simulink model "step3"  (R2018a)
settings: Solver=ode45  StartTime=0.0  StopTime=4  RelTol=1e-3
values from neighbouring files (symbols this model uses):
  Beta = 0    [step2.m]
  Friction = 22600    [step2.m]
  Inertia = 250000    [step2.m]
  Lambdam = 14.3522    [step2.m]
  Ld = 0.0035218    [step2.m]
  Lq = 0.0035218    [step2.m]
  Pole = 118    [step2.m]
  R = 58    [step2.m]
  Ro = 1.225    [step2.m]
  Rs = 0.05    [step2.m]
  Vw = 11.8    [step2.m]
undefined symbols (not defined in the file or in its folder): Cpmax, Lambda_opt, level, Ls, Ts
libraries: powerlib x18, peRmsMeasurement x8, peTransforms x2, simulink x2, powerlib_extras x1, simulink_extras x1
settings Model: Creator=Xinyi Zhang  LastModifiedBy=Xinyi Zhang

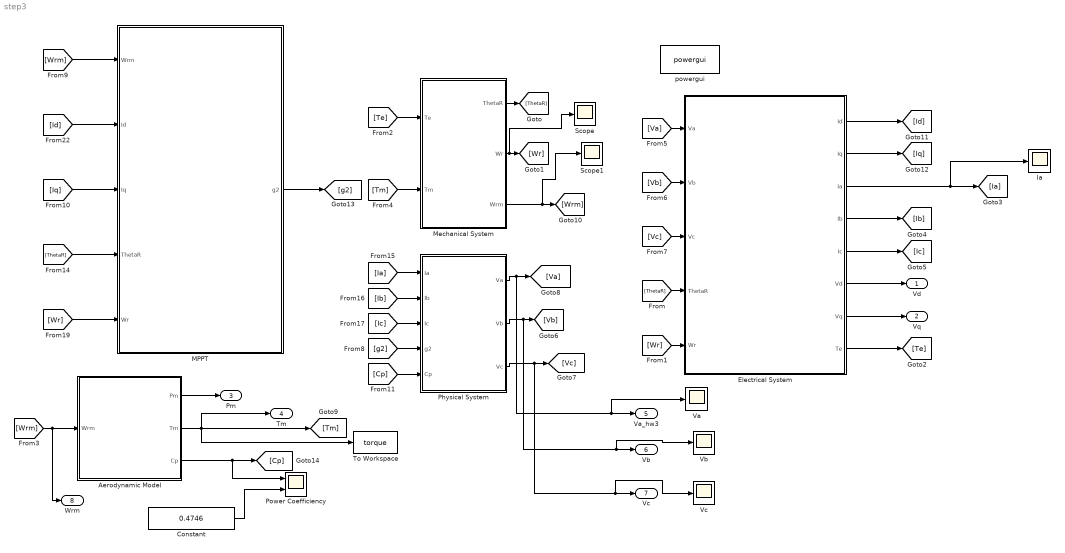
== system step3 ==
  "Aerodynamic Model " : Subsystem
  Constant : Constant  Value=0.4746
  "Electrical System " : Subsystem
  Ia : Scope
  "MPPT " : Subsystem
  "Mechanical System " : Subsystem
  "Physical System " : Subsystem
  "Power Coefficiency " : Scope  NumInputPorts=2
  Scope : Scope
  Scope1 : Scope
  To Workspace : ToWorkspace  VariableName=torque  SaveFormat=Timeseries  SampleTime=-1
  "Va " : Scope
  Vb : Scope
  Vc : Scope
  powergui : powerlib/powergui  Priority=1  SimulationMode=Discrete  SampleTime=25e-6  frequency=60  Iterations=50  frequencyindice=0  Pbase=100e6  ErrMax=1e-4  UnitsV=kV  UnitsW=MW  buscounter=0  FunctionMessages=off  echomessages=off  EnableUseOfTLC=off  CurrentSourceSwitches=off  DisableSnubberDevices=off  DisableRonSwitches=off  DisableVfSwitches=off  DisplayEquations=off  SolverType=Tustin/Backward Euler (TBE)  Interpol=off  ExternalGateDelay=off  methode=off  Ts=100  x0status=blocks  SPID=on  SwTol=0  HookPort=off  RestoreLinks=warning  ResistiveCurrentMeasurement=off  Frange=[0:2:500]  Ylog=off  Xlog=on  ShowGrid=off  save=off  variable=ZData  structure=0  ZoomFFT=off  StartTime=0.0  cycles=1  DisplayStyle=1  fundamental=60  FreqAxis=off  MaxFrequency=1000  frequencyindicesteady=1  RmsSteady=1  display=off
  "Vd " : Outport
  "Vq " : Outport  Port=2
  Pm : Outport  Port=3
  Tm : Outport  Port=4
  "Va_hw3 " : Outport  Port=5
  "Vb " : Outport  Port=6
  "Vc " : Outport  Port=7
  "Wrm " : Outport  Port=8
  wires:
  "Mechanical System "/1("ThetaR ") -> [ThetaR]
  [ThetaR] -> "Electrical System "/4(ThetaR)
  [Wr] -> "Electrical System "/5(Wr)
  [Va] -> "Electrical System "/1(Va)
  [Vb] -> "Electrical System "/2(Vb)
  [Vc] -> "Electrical System "/3(Vc)
  "Mechanical System "/2(Wr) -> Scope/1, [Wr]
  "Electrical System "/1(Id) -> [Id]
  "Electrical System "/2(Iq) -> [Iq]
  [Ia] -> "Physical System "/1("Ia ")
  [Ib] -> "Physical System "/2("Ib ")
  [Ic] -> "Physical System "/3("Ic ")
  "Physical System "/1("Va ") -> "Va "/1, "Va_hw3 "/1, [Va]
  "Physical System "/2("Vb ") -> Vb/1, "Vb "/1, [Vb]
  "Physical System "/3("Vc ") -> Vc/1, "Vc "/1, [Vc]
  [Te] -> "Mechanical System "/1(Te)
  "Electrical System "/4(Ib) -> [Ib]
  "Electrical System "/6("Vd ") -> "Vd "/1
  "Electrical System "/7("Vq ") -> "Vq "/1
  [Wrm] -> "Wrm "/1, "Aerodynamic Model "/1("Wrm ")
  "Aerodynamic Model "/1(Pm) -> Pm/1
  "Aerodynamic Model "/2(Tm) -> To Workspace/1, Tm/1, [Tm]
  "Mechanical System "/3("Wrm ") -> Scope1/1, [Wrm]
  "Electrical System "/3(Ia) -> Ia/1, [Ia]
  "Electrical System "/8("Te ") -> [Te]
  [Tm] -> "Mechanical System "/2("Tm ")
  "Electrical System "/5(Ic) -> [Ic]
  [g2] -> "Physical System "/4(g2)
  [Id] -> "MPPT "/2("Id ")
  [Wr] -> "MPPT "/5("Wr ")
  [ThetaR] -> "MPPT "/4("ThetaR ")
  [Iq] -> "MPPT "/3("Iq ")
  [Wrm] -> "MPPT "/1(Wrm)
  "MPPT "/1(g2) -> [g2]
  "Aerodynamic Model "/3("Cp ") -> "Power Coefficiency "/1, [Cp]
  [Cp] -> "Physical System "/5(Cp)
  Constant/1 -> "Power Coefficiency "/2

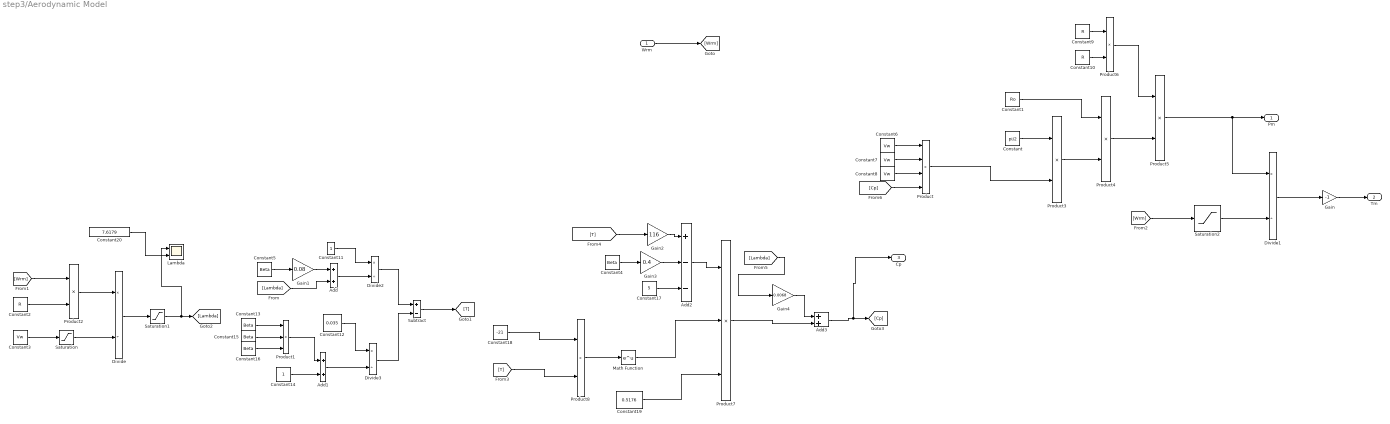
== system step3/Aerodynamic Model  ==
  "Wrm " : Inport
  Add : Sum
  Add1 : Sum
  Add2 : Sum  Inputs=+--
  Add3 : Sum
  Constant : Constant  Value=pi/2
  Constant1 : Constant  Value=Ro
  Constant10 : Constant  Value=R
  Constant11 : Constant
  Constant12 : Constant  Value=0.035
  Constant{4..5,13,15..16} (5 alike) : Constant  Value=Beta
  Constant14 : Constant
  Constant17 : Constant  Value=5
  Constant18 : Constant  Value=-21
  Constant19 : Constant  Value=0.5176
  Constant2 : Constant  Value=R
  Constant20 : Constant  Value=7.6179
  Constant{3,6..8} (4 alike) : Constant  Value=Vw
  Constant9 : Constant  Value=R
  Divide{,1..3} (4 alike) : Product  Inputs=*/
  Gain : Gain  Gain=-1
  Gain1 : Gain  Gain=0.08
  Gain2 : Gain  Gain=116
  Gain3 : Gain  Gain=0.4
  Gain4 : Gain  Gain=0.0068
  "Lambda " : Scope  NumInputPorts=2
  Math Function : Math  SaturateOnIntegerOverflow=on
  Product : Product  Inputs=4
  Product1 : Product  Inputs=3
  Product{2..6,8} (6 alike) : Product
  Product7 : Product  Inputs=3
  Saturation : Saturate  UpperLimit=1e6  LowerLimit=1e-6
  Saturation1 : Saturate  UpperLimit=1e6  LowerLimit=1e-6
  Saturation2 : Saturate  UpperLimit=1e6  LowerLimit=1e-6
  Subtract : Sum  Inputs=+-
  Pm : Outport
  Tm : Outport  Port=2
  "Cp " : Outport  Port=3
  wires:
  [Wrm] -> Product2/1
  "Wrm "/1 -> [Wrm]
  Product2/1 -> Divide/1
  Saturation/1 -> Divide/2
  Divide/1 -> Saturation1/1
  Constant/1 -> Product3/1
  Product3/1 -> Product4/2
  Constant1/1 -> Product4/1
  Product4/1 -> Product5/2
  Product6/1 -> Product5/1
  Product5/1 -> Divide1/1, Pm/1
  Saturation2/1 -> Divide1/2
  Divide1/1 -> Gain/1
  Gain/1 -> Tm/1
  Constant2/1 -> Product2/2
  Constant3/1 -> Saturation/1
  Constant8/1 -> Product/3
  Constant7/1 -> Product/2
  Constant6/1 -> Product/1
  Constant9/1 -> Product6/1
  Constant10/1 -> Product6/2
  Product/1 -> Product3/2
  [Wrm] -> Saturation2/1
  Constant5/1 -> Gain1/1
  Gain1/1 -> Add/1
  [Lambda] -> Add/2
  Add/1 -> Divide2/2
  Constant11/1 -> Divide2/1
  Add1/1 -> Divide3/2
  Product1/1 -> Add1/1
  Constant12/1 -> Divide3/1
  Constant14/1 -> Add1/2
  Constant13/1 -> Product1/1
  Constant15/1 -> Product1/2
  Constant16/1 -> Product1/3
  Divide2/1 -> Subtract/1
  Divide3/1 -> Subtract/2
  Subtract/1 -> [T]
  Saturation1/1 -> "Lambda "/1, [Lambda]
  Gain2/1 -> Add2/1
  [T] -> Gain2/1
  Constant4/1 -> Gain3/1
  Gain3/1 -> Add2/2
  Constant17/1 -> Add2/3
  Add2/1 -> Product7/1
  Math Function/1 -> Product7/2
  Constant19/1 -> Product7/3
  Product7/1 -> Add3/2
  [Lambda] -> Gain4/1
  Gain4/1 -> Add3/1
  Add3/1 -> "Cp "/1, [Cp]
  [Cp] -> Product/4
  Product8/1 -> Math Function/1
  Constant18/1 -> Product8/1
  [T] -> Product8/2
  Constant20/1 -> "Lambda "/2

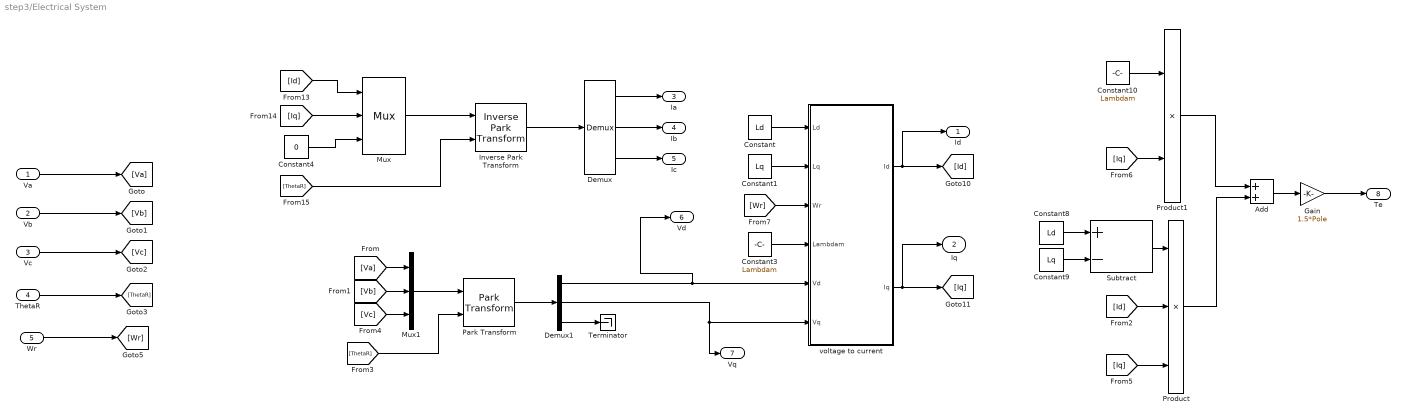
== system step3/Electrical System  ==
  Va : Inport
  Vb : Inport  Port=2
  Vc : Inport  Port=3
  ThetaR : Inport  Port=4
  Wr : Inport  Port=5
  Add : Sum
  Constant : Constant  Value=Ld
  Constant1 : Constant  Value=Lq
  Constant10 : Constant  Value=Lambdam
  Constant3 : Constant  Value=Lambdam
  Constant4 : Constant  Value=0
  Constant8 : Constant  Value=Ld
  Constant9 : Constant  Value=Lq
  Demux : Demux  Outputs=3
  Demux1 : Demux  Outputs=3
  Gain : Gain  Gain=1.5*Pole
  Inverse Park Transform : peTransforms/Inverse Park Transform  AxisAlignment=D-axis  PowerInvariant=off
  Mux : Mux  Inputs=3
  Mux1 : Mux  Inputs=3
  Park Transform : peTransforms/Park Transform  AxisAlignment=D-axis  PowerInvariant=off
  Product : Product  Inputs=3
  Product1 : Product
  Subtract : Sum  Inputs=+-
  Terminator : Terminator
  voltage to current : Subsystem
  Id : Outport
  Iq : Outport  Port=2
  Ia : Outport  Port=3
  Ib : Outport  Port=4
  Ic : Outport  Port=5
  "Vd " : Outport  Port=6
  "Vq " : Outport  Port=7
  "Te " : Outport  Port=8
  wires:
  Va/1 -> [Va]
  Vb/1 -> [Vb]
  Vc/1 -> [Vc]
  ThetaR/1 -> [ThetaR]
  Wr/1 -> [Wr]
  [Wr] -> voltage to current/3(Wr)
  Constant/1 -> voltage to current/1(Ld)
  Constant1/1 -> voltage to current/2("Lq ")
  Constant3/1 -> voltage to current/4(Lambdam)
  voltage to current/1(Id) -> Id/1, [Id]
  voltage to current/2(Iq) -> Iq/1, [Iq]
  [Id] -> Mux/1
  [Iq] -> Mux/2
  Constant4/1 -> Mux/3
  Demux/1 -> Ia/1
  Demux/2 -> Ib/1
  Demux/3 -> Ic/1
  [Va] -> Mux1/1
  [Vb] -> Mux1/2
  [Vc] -> Mux1/3
  Demux1/1 -> voltage to current/5("Vd "), "Vd "/1
  Demux1/2 -> "Vq "/1, voltage to current/6(Vq)
  Mux/1 -> Inverse Park Transform/1
  Inverse Park Transform/1 -> Demux/1
  [ThetaR] -> Inverse Park Transform/2
  Mux1/1 -> Park Transform/1
  [ThetaR] -> Park Transform/2
  Park Transform/1 -> Demux1/1
  Product/1 -> Add/2
  Add/1 -> Gain/1
  Product1/1 -> Add/1
  Constant9/1 -> Subtract/2
  Subtract/1 -> Product/1
  Gain/1 -> "Te "/1
  [Iq] -> Product/3
  Constant8/1 -> Subtract/1
  Constant10/1 -> Product1/1
  [Id] -> Product/2
  [Iq] -> Product1/2
  Demux1/3 -> Terminator/1

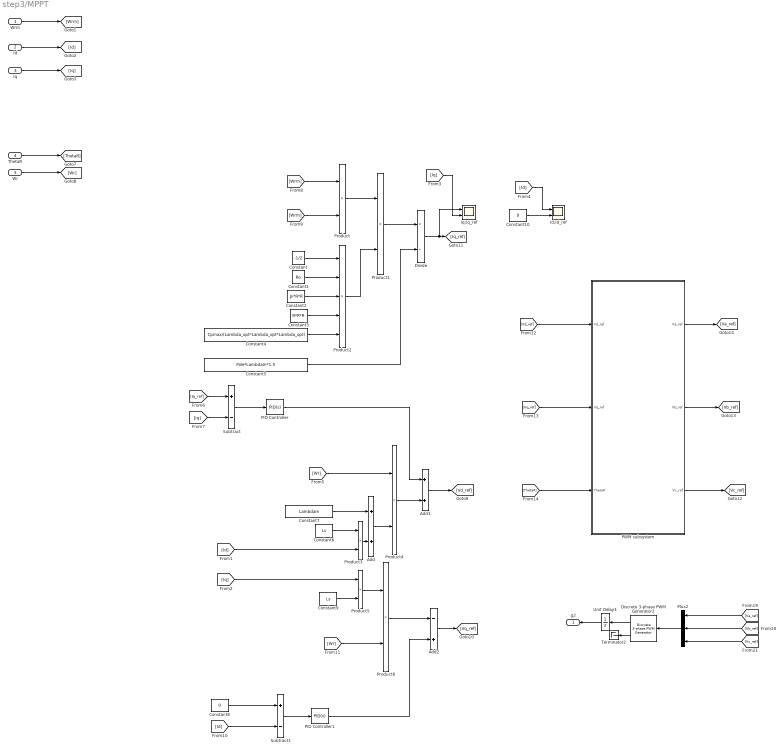
== system step3/MPPT  ==
  Wrm : Inport
  "Id " : Inport  Port=2
  "Iq " : Inport  Port=3
  "ThetaR " : Inport  Port=4
  "Wr " : Inport  Port=5
  Add : Sum
  Add1 : Sum
  Add2 : Sum  Inputs=-+
  Constant : Constant  Value=-1/2
  Constant1 : Constant  Value=Ro
  Constant10 : Constant  Value=0
  Constant2 : Constant  Value=pi*R*R
  Constant3 : Constant  Value=R*R*R
  Constant4 : Constant  Value=Cpmax/(Lambda_opt*Lambda_opt*Lambda_opt)
  Constant5 : Constant  Value=Pole*Lambdam*1.5
  Constant6 : Constant  Value=Ls
  Constant7 : Constant  Value=Lambdam
  Constant8 : Constant  Value=0
  Constant9 : Constant  Value=Ls
  Discrete 3-phase PWM Generator2 : powerlib_extras/Discrete  Control Blocks/Discrete 3-phase PWM Generator  ModulatorType=3-level  ModulatorMode=Un-synchronized  nF=18  Fc=2400  ModulatingSignals=off  m=0.2  Freq=60  Phase=0  Ts=Ts
  Divide : Product  Inputs=*/
  "Id;Id_ref " : Scope  NumInputPorts=2
  "Iq;Iq_ref " : Scope  NumInputPorts=2
  Mux2 : Mux  Inputs=3
  PID Controller : simulink/Continuous/PID Controller  Controller=PID  TimeDomain=Continuous-time  SampleTime=-1  IntegratorMethod=Forward Euler  FilterMethod=Forward Euler  Form=Parallel  UseFilter=on  ControllerParametersSource=internal  P=1  I=1  D=0  N=100  InitialConditionSource=internal  InitialConditionForIntegrator=0  InitialConditionForFilter=0  ExternalReset=none  LimitOutput=off  UpperSaturationLimit=inf  LowerSaturationLimit=-inf  LinearizeAsGain=on  AntiWindupMode=none  Kb=1  TrackingMode=off  Kt=1  PParamMin=[]  PParamMax=[]  IParamMin=[]  IParamMax=[]  DParamMin=[]  DParamMax=[]  NParamMin=[]  NParamMax=[]  KbParamMin=[]  KbParamMax=[]  KtParamMin=[]  KtParamMax=[]  POutMin=[]  POutMax=[]  IOutMin=[]  IOutMax=[]  DOutMin=[]  DOutMax=[]  NOutMin=[]  NOutMax=[]  KbOutMin=[]  KbOutMax=[]  KtOutMin=[]  KtOutMax=[]  IntegratorOutMin=[]  IntegratorOutMax=[]  FilterOutMin=[]  FilterOutMax=[]  SumOutMin=[]  SumOutMax=[]  SumI1OutMin=[]  SumI1OutMax=[]  SumI2OutMin=[]  SumI2OutMax=[]  SumI3OutMin=[]  SumI3OutMax=[]  SumDOutMin=[]  SumDOutMax=[]  SaturationOutMin=[]  SaturationOutMax=[]  IntegratorContinuousStateAttributes=''  IntegratorStateMustResolveToSignalObject=off  IntegratorRTWStateStorageClass=Auto  FilterContinuousStateAttributes=''  FilterStateMustResolveToSignalObject=off  FilterRTWStateStorageClass=Auto  DifferentiatorICPrevScaledInput=0  DifferentiatorOutMin=[]  DifferentiatorOutMax=[]  FilterDiffOutCoefMin=[]  FilterDiffOutCoefMax=[]  SumDenOutMin=[]  SumDenOutMax=[]  SumNumOutMin=[]  SumNumOutMax=[]  ReciprocalOutMin=[]  ReciprocalOutMax=[]  DivideOutMin=[]  DivideOutMax=[]  TunerSelectOption=Transfer Function Based (PID Tuner App)
  PID Controller1 : simulink/Continuous/PID Controller  Controller=PID  TimeDomain=Continuous-time  SampleTime=-1  IntegratorMethod=Forward Euler  FilterMethod=Forward Euler  Form=Parallel  UseFilter=on  ControllerParametersSource=internal  P=1  I=1  D=0  N=100  InitialConditionSource=internal  InitialConditionForIntegrator=0  InitialConditionForFilter=0  ExternalReset=none  LimitOutput=off  UpperSaturationLimit=inf  LowerSaturationLimit=-inf  LinearizeAsGain=on  AntiWindupMode=none  Kb=1  TrackingMode=off  Kt=1  PParamMin=[]  PParamMax=[]  IParamMin=[]  IParamMax=[]  DParamMin=[]  DParamMax=[]  NParamMin=[]  NParamMax=[]  KbParamMin=[]  KbParamMax=[]  KtParamMin=[]  KtParamMax=[]  POutMin=[]  POutMax=[]  IOutMin=[]  IOutMax=[]  DOutMin=[]  DOutMax=[]  NOutMin=[]  NOutMax=[]  KbOutMin=[]  KbOutMax=[]  KtOutMin=[]  KtOutMax=[]  IntegratorOutMin=[]  IntegratorOutMax=[]  FilterOutMin=[]  FilterOutMax=[]  SumOutMin=[]  SumOutMax=[]  SumI1OutMin=[]  SumI1OutMax=[]  SumI2OutMin=[]  SumI2OutMax=[]  SumI3OutMin=[]  SumI3OutMax=[]  SumDOutMin=[]  SumDOutMax=[]  SaturationOutMin=[]  SaturationOutMax=[]  IntegratorContinuousStateAttributes=''  IntegratorStateMustResolveToSignalObject=off  IntegratorRTWStateStorageClass=Auto  FilterContinuousStateAttributes=''  FilterStateMustResolveToSignalObject=off  FilterRTWStateStorageClass=Auto  DifferentiatorICPrevScaledInput=0  DifferentiatorOutMin=[]  DifferentiatorOutMax=[]  FilterDiffOutCoefMin=[]  FilterDiffOutCoefMax=[]  SumDenOutMin=[]  SumDenOutMax=[]  SumNumOutMin=[]  SumNumOutMax=[]  ReciprocalOutMin=[]  ReciprocalOutMax=[]  DivideOutMin=[]  DivideOutMax=[]  TunerSelectOption=Transfer Function Based (PID Tuner App)
  "PWM subsystem " : Subsystem
  Product{,1,3..6} (6 alike) : Product
  Product2 : Product  Inputs=5
  Subtract : Sum  Inputs=+-
  Subtract1 : Sum  Inputs=+-
  Terminator2 : Terminator
  Unit Delay3 : UnitDelay  SampleTime=Ts
  g2 : Outport
  wires:
  Product2/1 -> Product1/2
  [Wrm] -> Product/2
  Constant5/1 -> Divide/2
  Product1/1 -> Divide/1
  Constant1/1 -> Product2/2
  Constant2/1 -> Product2/3
  Product/1 -> Product1/1
  Divide/1 -> "Iq;Iq_ref "/1, [Iq_ref]
  Constant/1 -> Product2/1
  [Wrm] -> Product/1
  Constant3/1 -> Product2/4
  Constant4/1 -> Product2/5
  Wrm/1 -> [Wrm]
  "Id "/1 -> [Id]
  "Iq "/1 -> [Iq]
  "ThetaR "/1 -> [ThetaR]
  Constant6/1 -> Product3/1
  Product3/1 -> Add/2
  Constant7/1 -> Add/1
  Add/1 -> Product4/2
  [Wr] -> Product4/1
  "Wr "/1 -> [Wr]
  Product4/1 -> Add1/2
  [Iq_ref] -> Subtract/1
  [Iq] -> Subtract/2
  Subtract/1 -> PID Controller/1
  PID Controller/1 -> Add1/1
  [Id] -> Subtract1/2
  Constant8/1 -> Subtract1/1
  Subtract1/1 -> PID Controller1/1
  Constant9/1 -> Product5/2
  Product5/1 -> Product6/1
  [Wr] -> Product6/2
  Product6/1 -> Add2/1
  PID Controller1/1 -> Add2/2
  Add1/1 -> [Vd_ref]
  Add2/1 -> [Vq_ref]
  [Vd_ref] -> "PWM subsystem "/1("Vd_ref ")
  [Vq_ref] -> "PWM subsystem "/2("Vq_ref ")
  [ThetaR] -> "PWM subsystem "/3("ThetaR ")
  "PWM subsystem "/3("Vc_ref ") -> [Vc_ref]
  "PWM subsystem "/2("Vb_ref ") -> [Vb_ref]
  "PWM subsystem "/1("Va_ref ") -> [Va_ref]
  Discrete 3-phase PWM Generator2/2 -> Terminator2/1
  Discrete 3-phase PWM Generator2/1 -> Unit Delay3/1
  Mux2/1 -> Discrete 3-phase PWM Generator2/1
  [Va_ref] -> Mux2/1
  [Vb_ref] -> Mux2/2
  [Vc_ref] -> Mux2/3
  Unit Delay3/1 -> g2/1
  [Id] -> Product3/2
  [Iq] -> Product5/1
  [Iq] -> "Iq;Iq_ref "/2
  [Id] -> "Id;Id_ref "/1
  Constant10/1 -> "Id;Id_ref "/2

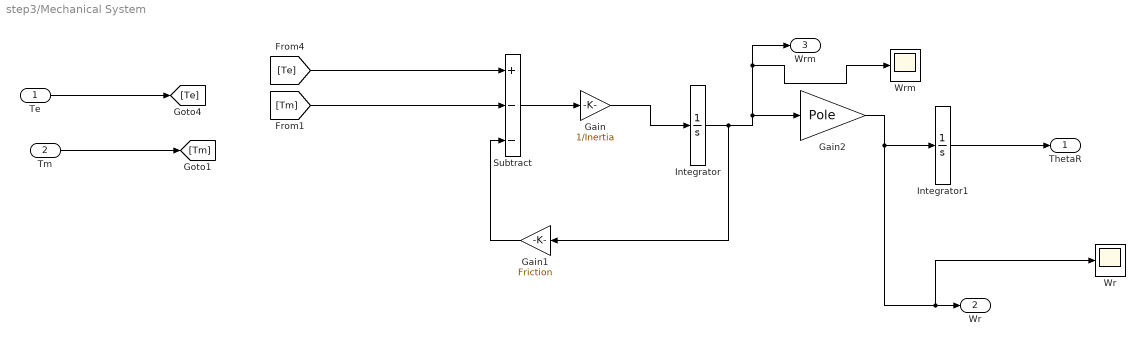
== system step3/Mechanical System  ==
  Te : Inport
  "Tm " : Inport  Port=2
  Gain : Gain  Gain=1/Inertia
  Gain1 : Gain  Gain=Friction
  Gain2 : Gain  Gain=Pole
  Integrator : Integrator
  Integrator1 : Integrator
  Subtract : Sum  Inputs=+--
  "Wr " : Scope
  Wrm : Scope
  "ThetaR " : Outport
  Wr : Outport  Port=2
  "Wrm " : Outport  Port=3
  wires:
  Integrator1/1 -> "ThetaR "/1
  Gain2/1 -> "Wr "/1, Wr/1, Integrator1/1
  Integrator/1 -> Wrm/1, "Wrm "/1, Gain2/1, Gain1/1
  [Te] -> Subtract/1
  Te/1 -> [Te]
  Subtract/1 -> Gain/1
  Gain/1 -> Integrator/1
  Gain1/1 -> Subtract/3
  "Tm "/1 -> [Tm]
  [Tm] -> Subtract/2

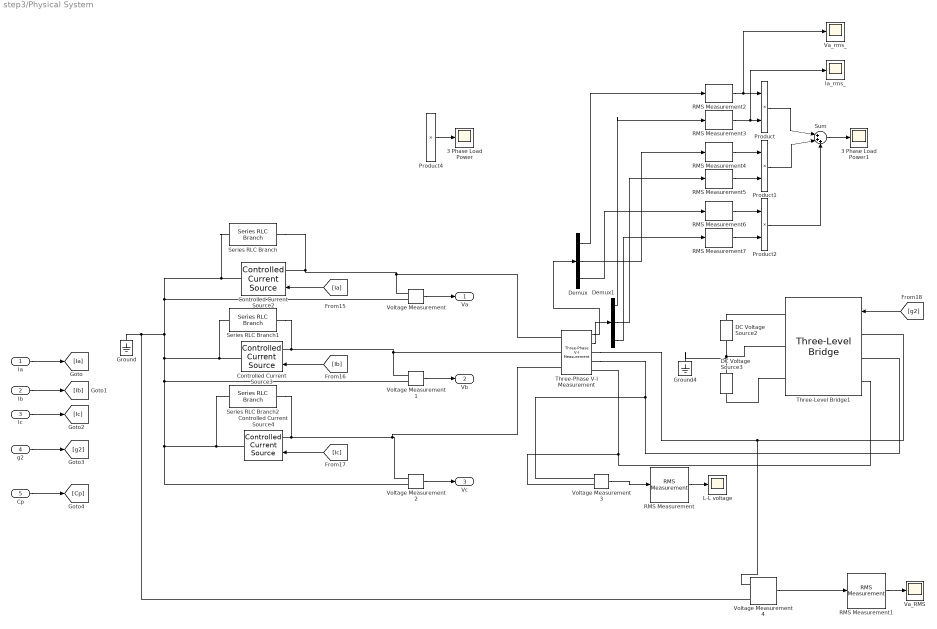
== system step3/Physical System  ==
  "Ia " : Inport
  "Ib " : Inport  Port=2
  "Ic " : Inport  Port=3
  g2 : Inport  Port=4
  Cp : Inport  Port=5
  3 Phase Load Power : Scope
  3 Phase Load Power1 : Scope
  Controlled Current Source2 : powerlib/Electrical Sources/Controlled Current Source  Initialize=on  Source_Type=AC  Amplitude=0  Phase=0  Frequency=0  Measurements=None
  Controlled Current Source3 : powerlib/Electrical Sources/Controlled Current Source  Initialize=on  Source_Type=AC  Amplitude=0  Phase=0  Frequency=0  Measurements=None
  Controlled Current Source4 : powerlib/Electrical Sources/Controlled Current Source  Initialize=on  Source_Type=AC  Amplitude=0  Phase=0  Frequency=0  Measurements=None
  DC Voltage Source2 : powerlib/Electrical Sources/DC Voltage Source  Amplitude=2500  Measurements=None
  DC Voltage Source3 : powerlib/Electrical Sources/DC Voltage Source  Amplitude=2500  Measurements=None
  Demux : Demux  Outputs=3
  Demux1 : Demux  Outputs=3
  Ground : powerlib/Elements/Ground  LConnTagsString=a
  Ground4 : powerlib/Elements/Ground  LConnTagsString=a
  Ia_rms_ : Scope
  L-L voltage : Scope
  Product{,1..2,4} (4 alike) : Product
  RMS Measurement{,1..7} (8 alike) : peRmsMeasurement/RMS Measurement  OverrideUsingVariant=Total  F=60  SpecifyHarmonics=off  K=[0 1 2]  Ts=0
  Series RLC Branch : powerlib/Elements/Series RLC Branch  LConnTagsString=__new0  RConnTagsString=__new0  BranchType=R  Resistance=1000000  Inductance=1e-3  SetiL0=off  InitialCurrent=0  Capacitance=1e-6  Setx0=off  InitialVoltage=0  Measurements=None
  Series RLC Branch1 : powerlib/Elements/Series RLC Branch  LConnTagsString=__new0  RConnTagsString=__new0  BranchType=R  Resistance=1000000  Inductance=1e-3  SetiL0=off  InitialCurrent=0  Capacitance=1e-6  Setx0=off  InitialVoltage=0  Measurements=None
  Series RLC Branch2 : powerlib/Elements/Series RLC Branch  LConnTagsString=__new0  RConnTagsString=__new0  BranchType=R  Resistance=1000000  Inductance=1e-3  SetiL0=off  InitialCurrent=0  Capacitance=1e-6  Setx0=off  InitialVoltage=0  Measurements=None
  Sum : Sum  Inputs=|+++
  Three-Level Bridge1 : powerlib/Power Electronics/Three-Level Bridge  Arms=3  SnubberResistance=1e3  SbubberCapacitance=1e-6  Device=Ideal Switches  Ron=0.2e-3  ForwardVoltages="[  2 1 ]"  Measurements=None
      settings: SourceProductName=Simscape Power Systems  SourceProductBaseCode=PS
  Three-Phase V-I Measurement : powerlib/Measurements/Three-Phase V-I Measurement  VoltageMeasurement=phase-to-ground  SetLabelV=off  LabelV=Vabc  Vpu=off  VpuLL=off  CurrentMeasurement=yes  SetLabelI=off  LabelI=Iabc  Ipu=off  Pbase=100e6  Vbase=500e3  OutputType=Complex  PhasorSimulation=off  PSBequivalent=0
  "Va_RMS " : Scope
  Va_rms_ : Scope
  Voltage Measurement{,1..4} (5 alike) : powerlib/Measurements/Voltage Measurement  PhasorSimulation=off  OutputType=Complex  PSBequivalent=0
  "Va " : Outport
  "Vb " : Outport  Port=2
  "Vc " : Outport  Port=3
  wires:
  [Ib] -> Controlled Current Source3/1
  [Ia] -> Controlled Current Source2/1
  [Ic] -> Controlled Current Source4/1
  "Ia "/1 -> [Ia]
  "Ib "/1 -> [Ib]
  "Ic "/1 -> [Ic]
  Voltage Measurement1/1 -> "Vb "/1
  Voltage Measurement2/1 -> "Vc "/1
  Voltage Measurement/1 -> "Va "/1
  [g2] -> Three-Level Bridge1/1
  g2/1 -> [g2]
  RMS Measurement/1 -> L-L voltage/1
  Voltage Measurement3/1 -> RMS Measurement/1
  Product/1 -> Sum/1
  Cp/1 -> [Cp]
  Product4/1 -> 3 Phase Load Power/1
  RMS Measurement1/1 -> "Va_RMS "/1
  Voltage Measurement4/1 -> RMS Measurement1/1
  Three-Phase V-I Measurement/1 -> Demux/1
  Three-Phase V-I Measurement/2 -> Demux1/1
  Sum/1 -> 3 Phase Load Power1/1
  RMS Measurement2/1 -> Va_rms_/1, Product/1
  RMS Measurement4/1 -> Product1/1
  RMS Measurement6/1 -> Product2/1
  Product1/1 -> Sum/2
  Product2/1 -> Sum/3
  Demux/1 -> RMS Measurement2/1
  Demux1/1 -> RMS Measurement3/1
  Demux/2 -> RMS Measurement4/1
  Demux1/2 -> RMS Measurement5/1
  Demux/3 -> RMS Measurement6/1
  Demux1/3 -> RMS Measurement7/1
  RMS Measurement7/1 -> Product2/2
  RMS Measurement3/1 -> Ia_rms_/1, Product/2
  RMS Measurement5/1 -> Product1/2
  connections:
  Controlled Current Source2/RConn1 -- Series RLC Branch/LConn1 -- Voltage Measurement2/LConn2 -- Series RLC Branch2/LConn1 -- Controlled Current Source4/RConn1 -- Voltage Measurement1/LConn2 -- Series RLC Branch1/LConn1 -- Controlled Current Source3/RConn1 -- Voltage Measurement4/LConn2 -- Ground/LConn1 -- Voltage Measurement/LConn2
  Series RLC Branch/RConn1 -- Three-Phase V-I Measurement/LConn1 -- Voltage Measurement/LConn1 -- Controlled Current Source2/LConn1
  Series RLC Branch1/RConn1 -- Three-Phase V-I Measurement/LConn2 -- Voltage Measurement1/LConn1 -- Controlled Current Source3/LConn1
  Series RLC Branch2/RConn1 -- Three-Phase V-I Measurement/LConn3 -- Voltage Measurement2/LConn1 -- Controlled Current Source4/LConn1
  DC Voltage Source3/RConn1 -- Ground4/LConn1 -- Three-Level Bridge1/RConn2 -- DC Voltage Source2/LConn1
  Three-Level Bridge1/RConn1 -- DC Voltage Source2/RConn1
  Three-Level Bridge1/RConn3 -- DC Voltage Source3/LConn1
  Three-Phase V-I Measurement/RConn1 -- Voltage Measurement4/LConn1 -- Three-Level Bridge1/LConn1
  Three-Phase V-I Measurement/RConn2 -- Voltage Measurement3/LConn1 -- Three-Level Bridge1/LConn2
  Three-Level Bridge1/LConn3 -- Voltage Measurement3/LConn2 -- Three-Phase V-I Measurement/RConn3

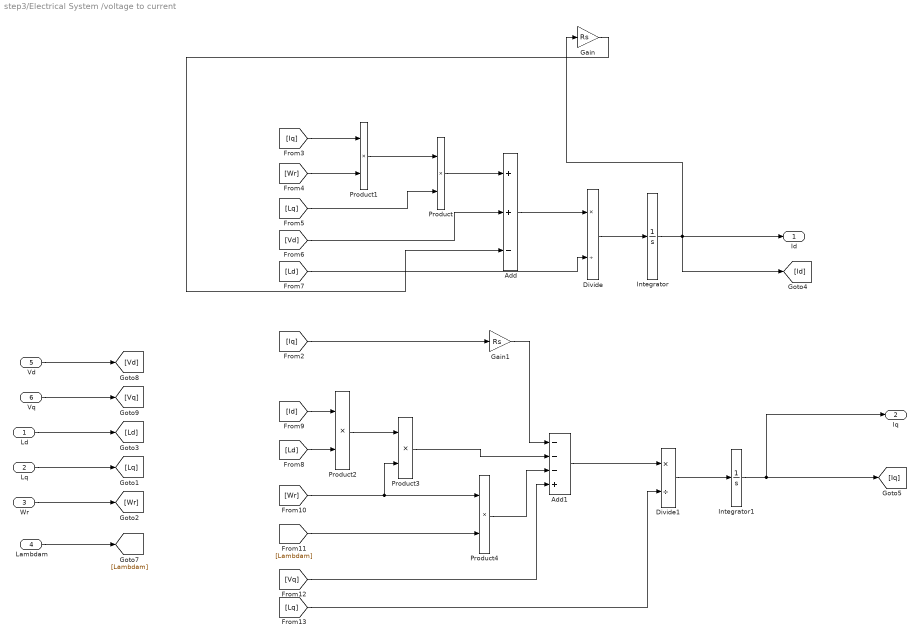
== system step3/Electrical System /voltage to current ==
  Ld : Inport
  "Lq " : Inport  Port=2
  Wr : Inport  Port=3
  Lambdam : Inport  Port=4
  "Vd " : Inport  Port=5
  Vq : Inport  Port=6
  Add : Sum  Inputs=++-
  Add1 : Sum  Inputs=---+
  Divide : Product  Inputs=*/
  Divide1 : Product  Inputs=*/
  Gain : Gain  Gain=Rs
  Gain1 : Gain  Gain=Rs
  Integrator : Integrator
  Integrator1 : Integrator
  Product{,1..4} (5 alike) : Product
  Id : Outport
  Iq : Outport  Port=2
  wires:
  Integrator/1 -> [Id], Gain/1, Id/1
  [Wr] -> Product3/2, Product4/1
  Product2/1 -> Product3/1
  Product1/1 -> Product/1
  Divide1/1 -> Integrator1/1
  Add/1 -> Divide/1
  [Id] -> Product2/1
  [Lambdam] -> Product4/2
  Divide/1 -> Integrator/1
  Integrator1/1 -> Iq/1, [Iq]
  [Iq] -> Product1/1
  [Wr] -> Product1/2
  [Lq] -> Product/2
  [Ld] -> Divide/2
  Product3/1 -> Add1/2
  [Vd] -> Add/2
  Add1/1 -> Divide1/1
  [Lq] -> Divide1/2
  [Ld] -> Product2/2
  Product/1 -> Add/1
  Product4/1 -> Add1/3
  [Vq] -> Add1/4
  Wr/1 -> [Wr]
  Ld/1 -> [Ld]
  "Lq "/1 -> [Lq]
  Lambdam/1 -> [Lambdam]
  "Vd "/1 -> [Vd]
  Vq/1 -> [Vq]
  Gain/1 -> Add/3
  [Iq] -> Gain1/1
  Gain1/1 -> Add1/1

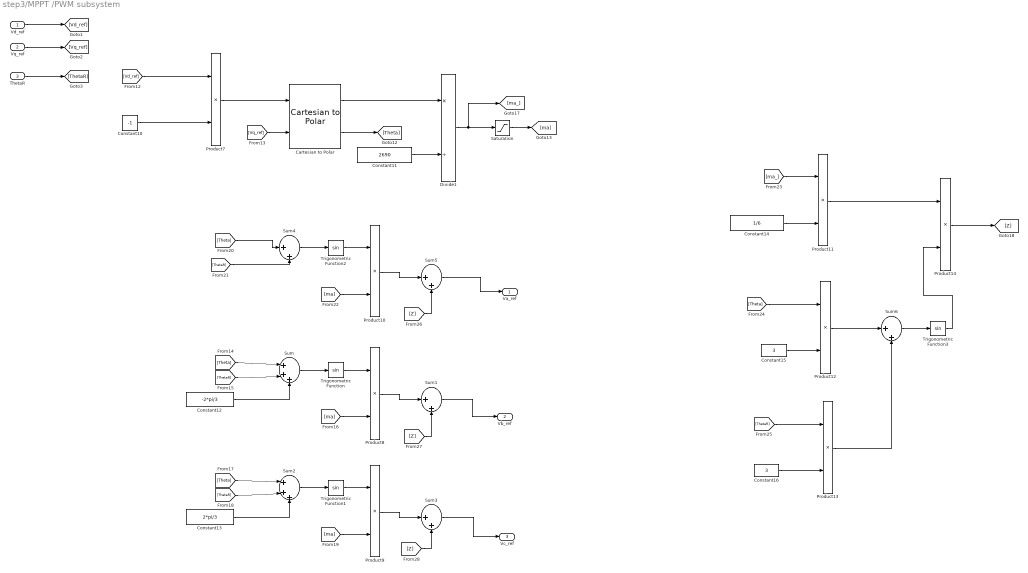
== system step3/MPPT /PWM subsystem  ==
  "Vd_ref " : Inport
  "Vq_ref " : Inport  Port=2
  "ThetaR " : Inport  Port=3
  Cartesian to Polar : simulink_extras/Transformations/Cartesian to Polar
      settings: SourceProductName=Simulink
  Constant10 : Constant  Value=-1
  Constant11 : Constant  Value=2690
  Constant12 : Constant  Value=-2*pi/3
  Constant13 : Constant  Value=2*pi/3
  Constant14 : Constant  Value=1/6
  Constant15 : Constant  Value=3
  Constant16 : Constant  Value=3
  Divide1 : Product  Inputs=*/
  Product{7..14} (8 alike) : Product
  Saturation : Saturate  UpperLimit=1.15  LowerLimit=0
  Sum : Sum  Inputs=|+++
  Sum{1,3..6} (5 alike) : Sum  Inputs=|++
  Sum2 : Sum  Inputs=|+++
  Trigonometric Function{,1..3} (4 alike) : Trigonometry
  "Va_ref " : Outport
  "Vb_ref " : Outport  Port=2
  "Vc_ref " : Outport  Port=3
  wires:
  [Z] -> Sum3/2
  [Vq_ref] -> Cartesian to Polar/2
  [ma_] -> Product11/1
  [ThetaR] -> Sum/2
  Constant12/1 -> Sum/3
  Product10/1 -> Sum5/1
  [Vd_ref] -> Product7/1
  [ThetaR] -> Product13/1
  Product7/1 -> Cartesian to Polar/1
  [Theta] -> Product12/1
  Sum2/1 -> Trigonometric Function1/1
  [Theta] -> Sum/1
  [ma] -> Product9/2
  Cartesian to Polar/1 -> Divide1/1
  [ma] -> Product8/2
  Product13/1 -> Sum6/2
  Sum6/1 -> Trigonometric Function3/1
  Constant13/1 -> Sum2/3
  [Z] -> Sum1/2
  Constant15/1 -> Product12/2
  Constant16/1 -> Product13/2
  Product9/1 -> Sum3/1
  Saturation/1 -> [ma]
  Trigonometric Function2/1 -> Product10/1
  Divide1/1 -> [ma_], Saturation/1
  Cartesian to Polar/2 -> [Theta]
  Sum/1 -> Trigonometric Function/1
  Product12/1 -> Sum6/1
  Product14/1 -> [Z]
  Trigonometric Function3/1 -> Product14/2
  Constant14/1 -> Product11/2
  [Z] -> Sum5/2
  Constant11/1 -> Divide1/2
  Sum3/1 -> "Vc_ref "/1
  Trigonometric Function1/1 -> Product9/1
  [Theta] -> Sum2/1
  [ThetaR] -> Sum2/2
  Product11/1 -> Product14/1
  Sum4/1 -> Trigonometric Function2/1
  Sum5/1 -> "Va_ref "/1
  [ThetaR] -> Sum4/2
  Constant10/1 -> Product7/2
  [Theta] -> Sum4/1
  [ma] -> Product10/2
  Sum1/1 -> "Vb_ref "/1
  Trigonometric Function/1 -> Product8/1
  Product8/1 -> Sum1/1
  "Vd_ref "/1 -> [Vd_ref]
  "Vq_ref "/1 -> [Vq_ref]
  "ThetaR "/1 -> [ThetaR]
